simulink model "nuri3s_Open_Loop_Model"  (R2024b)
settings: Solver=VariableStepAuto  StartTime=0.0  StopTime=10.0  RelTol=1e-3
undefined symbols (not defined in the file): timepoints, waypoints
libraries: robotmaniplib x2, robotcorelib x1
settings Model: Creator=user  LastModifiedBy=leeyh

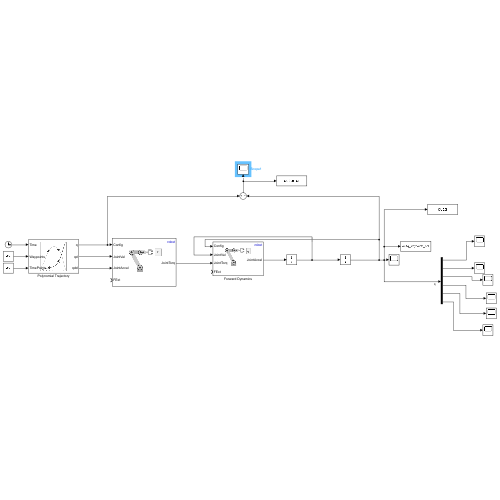
[thumbnail: Simulink's stored preview of the top-level diagram]
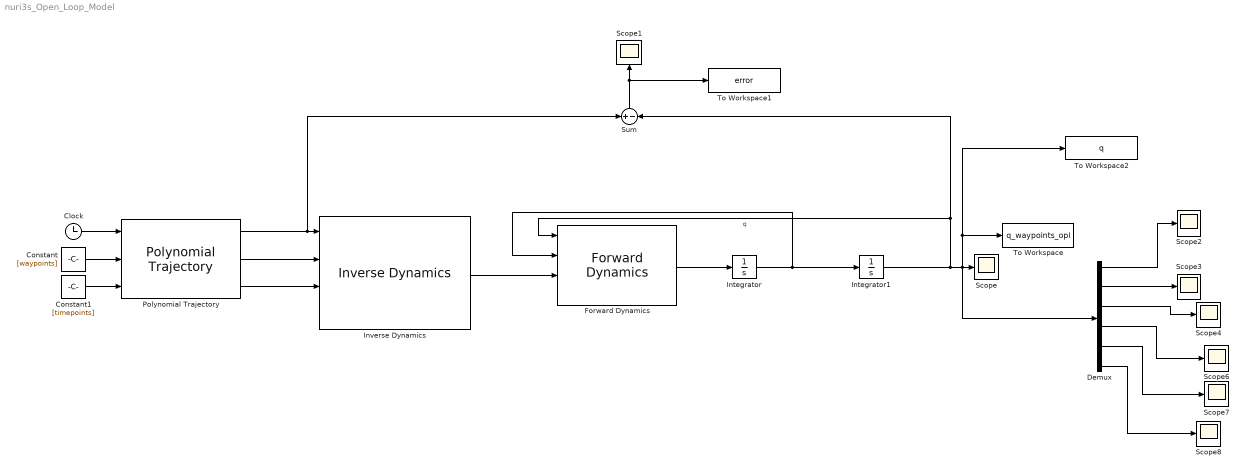
== system nuri3s_Open_Loop_Model ==
  Clock : Clock
  Constant : Constant  Value=[waypoints]
  Constant1 : Constant  Value=[timepoints]
  Demux : Demux  Outputs=6
  Forward Dynamics : robotmaniplib/Forward Dynamics  RigidBodyTree=robot  SimulateUsing=Interpreted execution
  Integrator : Integrator  InitialCondition=[0 0 -1.57 0 -1.57 0]
  Integrator1 : Integrator  InitialCondition=[0 0 -1.57 0 -1.57 0]
  Inverse Dynamics : robotmaniplib/Inverse Dynamics  RigidBodyTree=robot  SimulateUsing=Interpreted execution
  Polynomial Trajectory : robotcorelib/Polynomial Trajectory  WaypointSource=External  Waypoints=[ 0, 2, 1, 5, 0; -1, 3, 1, 4, 4 ]  TimePoints=[ 0, 1, 2, 3, 4 ]  TimeInterval=[ 1, 4 ]  Method=Quintic Polynomial  ParameterSource=Internal  VelocityBoundaryCondition=zeros( 6,100 )  AccelerationBoundaryCondition=zeros( 6,100 )  SimulateUsing=Interpreted execution
  Scope{,1..4,6..8} (8 alike) : Scope
  Sum : Sum  Inputs=+|-
  To Workspace : ToWorkspace  VariableName=q_waypoints_opl  SampleTime=-1
  To Workspace1 : ToWorkspace  VariableName=error  SaveFormat=Structure With Time  SampleTime=-1
  To Workspace2 : ToWorkspace  VariableName=q  SaveFormat=Structure With Time  SampleTime=-1
  wires:
  Forward Dynamics/1 -> Integrator/1
  Integrator/1 -> Forward Dynamics/2, Integrator1/1
  Polynomial Trajectory/1 -> Sum/1, Inverse Dynamics/1
  Polynomial Trajectory/2 -> Inverse Dynamics/2
  Polynomial Trajectory/3 -> Inverse Dynamics/3
  Inverse Dynamics/1 -> Forward Dynamics/3
  Clock/1 -> Polynomial Trajectory/1
  Constant/1 -> Polynomial Trajectory/2
  Constant1/1 -> Polynomial Trajectory/3
  Sum/1 -> To Workspace1/1, Scope1/1
  Demux/5 -> Scope7/1
  Demux/4 -> Scope6/1
  Demux/2 -> Scope3/1
  Integrator1/1 -> To Workspace/1, To Workspace2/1, Scope/1, Demux/1, Sum/2, Forward Dynamics/1  "q"
  Demux/3 -> Scope4/1
  Demux/6 -> Scope8/1
  Demux/1 -> Scope2/1
